simulink model "ereignis_zustand_umwandlung2"  (R2015b)
settings: Solver=FixedStepAuto  StartTime=0.0  StopTime=10.0  RelTol=1e-3
libraries: simulink x1
settings Model: Creator=scco1019  LastModifiedBy=scco1019

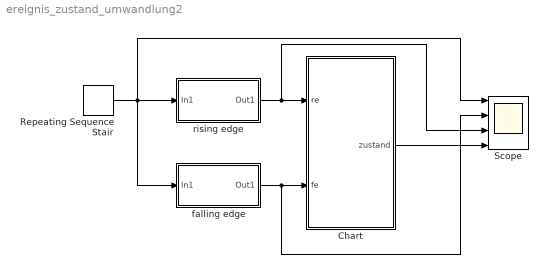
== system ereignis_zustand_umwandlung2 ==
  Chart : Stateflow chart  TreatAsAtomicUnit=on
  Repeating Sequence Stair : simulink/Sources/Repeating Sequence Stair  OutValues=[0 0 1 1 2 2 3 3 4 4 5 5 3 3 4 4 0 0]  tsamp=-1  OutMin=[]  OutMax=[]  OutDataTypeStr=double  OutputDataTypeScalingMode=double  OutDataType=fixdt(0,8)  ConRadixGroup=Best Precision: Vector-wise  OutScaling=2^-12
  Scope : Scope  NumInputPorts=4
  falling edge : Subsystem
  rising edge : Subsystem
  wires:
  Repeating Sequence Stair/1 -> falling edge/1(In1), rising edge/1(In1), Scope/1
  rising edge/1(Out1) -> Scope/3, Chart/1(re)
  falling edge/1(Out1) -> Scope/2, Chart/2(fe)
  Chart/1(zustand) -> Scope/4

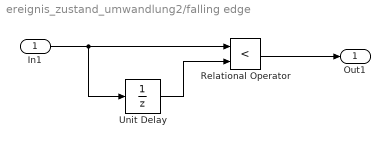
== system ereignis_zustand_umwandlung2/falling edge ==
  In1 : Inport
  Relational Operator : RelationalOperator  Operator=<  OutDataTypeStr=boolean
  Unit Delay : UnitDelay  SampleTime=-1
  Out1 : Outport
  wires:
  Unit Delay/1 -> Relational Operator/2
  Relational Operator/1 -> Out1/1
  In1/1 -> Unit Delay/1, Relational Operator/1

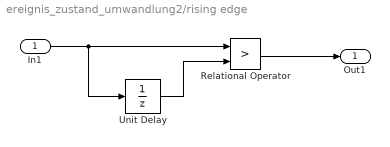
== system ereignis_zustand_umwandlung2/rising edge ==
  In1 : Inport
  Relational Operator : RelationalOperator  Operator=>  OutDataTypeStr=boolean
  Unit Delay : UnitDelay  SampleTime=-1
  Out1 : Outport
  wires:
  Unit Delay/1 -> Relational Operator/2
  Relational Operator/1 -> Out1/1
  In1/1 -> Unit Delay/1, Relational Operator/1

== stateflow chart ereignis_zustand_umwandlung2/Chart ==
  state Zustand_0/
    entry: zustand=0;
  state Zustand_1/
    entry: zustand=1;
  (default) -> Zustand_0
  Zustand_0 -> Zustand_0 [order 2]
  Zustand_1 -> Zustand_0 [order 1] : [fe==1]
  Zustand_0 -> Zustand_1 [order 1] : [re==1]
  Zustand_1 -> Zustand_1 [order 2]
  data: zustand output; re input; fe input
